simulink model "g4_regulated_converter"  (R2017a)
settings: Solver=ode23tb  StartTime=0  StopTime=1  RelTol=1e-3  EnableMultiTasking=on
undefined symbols (not defined in the file or in its folder): sigbuilder_block
libraries: powerlib x12, powerlib_meascontrol x1
settings Model: Creator=SHAKIL  LastModifiedBy=user
settings OptimizationCC: LifeSpan=inf
settings DebuggingCC: SFUnexpectedBacktrackingDiag=warning  SFNoUnconditionalDefaultTransitionDiag=warning  SFExecutionAtInitializationDiag=none
settings HardwareCC: ProdBitPerSizeT=32  ProdBitPerPtrDiffT=32  ProdWordSize=32  ProdHWDeviceType=Specified
settings GRTTargetCC: TargetLangStandard=C89/C90 (ANSI)  GeneratePreprocessorConditionals=Disable all
settings ConfigComp: CovMetricSettings=dw  CovHtmlReporting=on  CovSaveCumulativeToWorkspaceVar=on  CovSaveSingleToWorkspaceVar=on  CovExternalEMLEnable=off

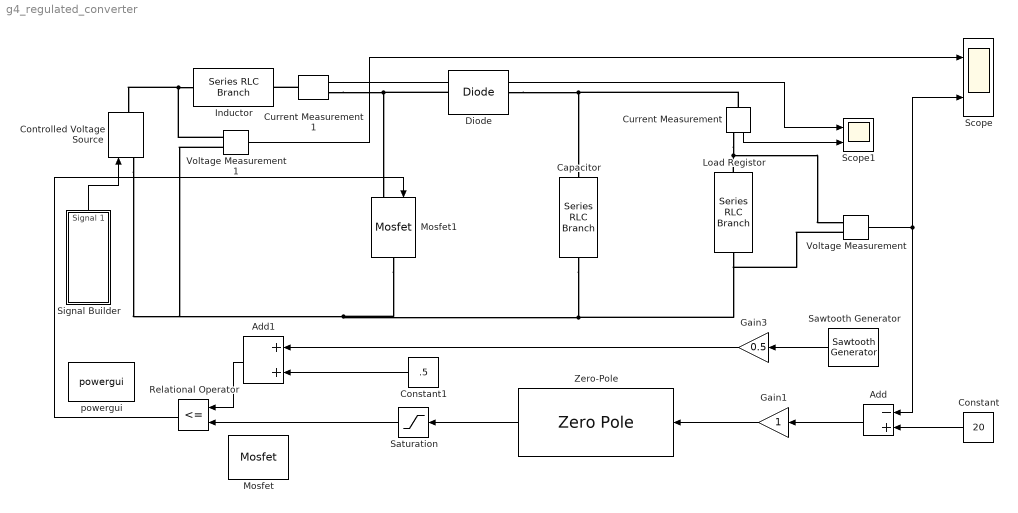
== system g4_regulated_converter ==
  Add : Sum  Inputs=-+
  Add1 : Sum
  Capacitor : powerlib/Elements/Series RLC Branch  LConnTagsString=__new0  RConnTagsString=__new0  BranchType=C  Resistance=1  Inductance=1e-3  SetiL0=off  InitialCurrent=0  Capacitance=78e-6  Setx0=off  InitialVoltage=0  Measurements=None
  Constant : Constant  Value=20
  Constant1 : Constant  Value=.5
  Controlled Voltage Source : powerlib/Electrical Sources/Controlled Voltage Source  Initialize=on  Source_Type=DC  Amplitude=0  Phase=0  Frequency=0  Measurements=None
  Current Measurement : powerlib/Measurements/Current Measurement  PhasorSimulation=off  OutputType=Complex  PSBequivalent=0
  Current Measurement1 : powerlib/Measurements/Current Measurement  PhasorSimulation=off  OutputType=Complex  PSBequivalent=0
  Diode : powerlib/Power Electronics/Diode  Ron=1e-9  Lon=0  Vf=0.1  IC=0  UseSnubber=off  Rs=0  Cs=0  Measurements=off
  Gain1 : Gain
  Gain3 : Gain  Gain=0.5
  Inductor : powerlib/Elements/Series RLC Branch  LConnTagsString=__new0  RConnTagsString=__new0  BranchType=L  Resistance=1  Inductance=35e-6  SetiL0=on  InitialCurrent=0  Capacitance=1e-6  Setx0=off  InitialVoltage=0  Measurements=None
  Load Registor : powerlib/Elements/Series RLC Branch  LConnTagsString=__new0  RConnTagsString=__new0  BranchType=R  Resistance=4  Inductance=1e-3  SetiL0=off  InitialCurrent=0  Capacitance=1e-6  Setx0=off  InitialVoltage=0  Measurements=None
  Mosfet : powerlib/Power Electronics/Mosfet  Ron=0.1  Lon=0  Rd=0.01  Vfd=0  IC=0  Rs=1e5  Cs=inf  Measurements=on
  Mosfet1 : powerlib/Power Electronics/Mosfet  Ron=0.1  Lon=0  Rd=0.01  Vfd=0  IC=0  Rs=1e5  Cs=inf  Measurements=off
  Relational Operator : RelationalOperator  Operator=<=  OutDataTypeStr=boolean  RndMeth=Nearest
  Saturation : Saturate  UpperLimit=0.6  LowerLimit=0.1
  Sawtooth Generator : powerlib_meascontrol/Pulse & Signal Generators/Sawtooth Generator  Freq=80e3  Phase=180  Ts=0
      settings: SourceProductName=Simscape Power Systems
  Scope : Scope  NumInputPorts=2
  Scope1 : Scope  NumInputPorts=2
  Signal Builder : Subsystem  Tag=STV Subsys  LoadFcn=sigbuilder_block('load');  StartFcn=sigbuilder_block('start');  StopFcn=sigbuilder_block('stop');  ClipboardFcn=sigbuilder_block('clipboard');  mask(Sigbuilder block){tuvar=[0:10]}
      mask help: Simulink:masks:SigbuilderBlock_MD
      mask init:
      | if ~strcmp(get_param(bdroot(gcbh),'SimulationStatus'),'stopped') tuvar = sigbuilder_block('maskInit'); end
      settings: CopyFcn=sigbuilder_block('copy');  DeleteFcn=sigbuilder_block('delete');  ModelCloseFcn=sigbuilder_block('modelClose');  PreSaveFcn=sigbuilder_block('preSave');  PauseFcn=sigbuilder_block('pause');  ContinueFcn=sigbuilder_block('continue');  NameChangeFcn=sigbuilder_block('namechange');  OpenFcn=sigbuilder_block('open',[6 6 1008 506.25 ]);  CloseFcn=sigbuilder_block('close');
      mask Display: plot(0, 0, 100, 100,[2, 2, 32, 32, 2], [68, 8, 8, 68, 68],[32, 2], [38, 38], [32, 19, 2],[53, 60, 44], [32, 17, 17, 2],[16, 16, 31, 31]);txt = getActiveGroup(gcbh);text(2, 100, txt,'verticalAlignment', 'top');
  Voltage Measurement : powerlib/Measurements/Voltage Measurement  PhasorSimulation=off  OutputType=Complex  PSBequivalent=0
  Voltage Measurement1 : powerlib/Measurements/Voltage Measurement  PhasorSimulation=off  OutputType=Complex  PSBequivalent=0
  Zero-Pole : ZeroPole  Zeros=[-2000 -2000]  Poles=[0 -10000]  Gain=[0.04]
  powergui : powerlib/powergui  Priority=1  SimulationMode=Continuous  SampleTime=50e-6  frequency=60  Iterations=50  frequencyindice=0  Pbase=100e6  ErrMax=1e-4  UnitsV=kV  UnitsW=MW  buscounter=0  FunctionMessages=off  echomessages=off  EnableUseOfTLC=off  CurrentSourceSwitches=off  DisableSnubberDevices=off  DisableRonSwitches=off  DisableVfSwitches=off  DisplayEquations=off  SolverType=Tustin/Backward Euler (TBE)  Interpol=off  ExternalGateDelay=off  methode=off  Ts=10  x0status=blocks  SPID=off  SwTol=0  HookPort=off  RestoreLinks=warning  ResistiveCurrentMeasurement=off  Frange=[0:2:500]  Ylog=off  Xlog=on  ShowGrid=off  save=off  variable=ZData  structure=0  ZoomFFT=off  StartTime=0.0  cycles=1  DisplayStyle=1  fundamental=60  FreqAxis=off  MaxFrequency=1000  frequencyindicesteady=1  RmsSteady=1  display=off
  wires:
  Voltage Measurement/1 -> Scope/2, Add/1
  Constant/1 -> Add/2
  Add/1 -> Gain1/1
  Signal Builder/1(Signal 1) -> Controlled Voltage Source/1
  Gain1/1 -> Zero-Pole/1
  Gain3/1 -> Add1/1
  Sawtooth Generator/1 -> Gain3/1
  Constant1/1 -> Add1/2
  Add1/1 -> Relational Operator/1
  Zero-Pole/1 -> Saturation/1
  Saturation/1 -> Relational Operator/2
  Voltage Measurement1/1 -> Scope/1
  Relational Operator/1 -> Mosfet1/1
  Current Measurement/1 -> Scope1/2
  Current Measurement1/1 -> Scope1/1
  connections:
  Voltage Measurement/LConn2 -- Load Registor/RConn1 -- Voltage Measurement1/LConn2 -- Controlled Voltage Source/LConn1 -- Mosfet1/RConn1 -- Capacitor/RConn1
  Load Registor/LConn1 -- Current Measurement/RConn1 -- Voltage Measurement/LConn1
  Diode/RConn1 -- Current Measurement/LConn1 -- Capacitor/LConn1
  Voltage Measurement1/LConn1 -- Controlled Voltage Source/RConn1 -- Inductor/LConn1
  Current Measurement1/LConn1 -- Inductor/RConn1
  Current Measurement1/RConn1 -- Mosfet1/LConn1 -- Diode/LConn1

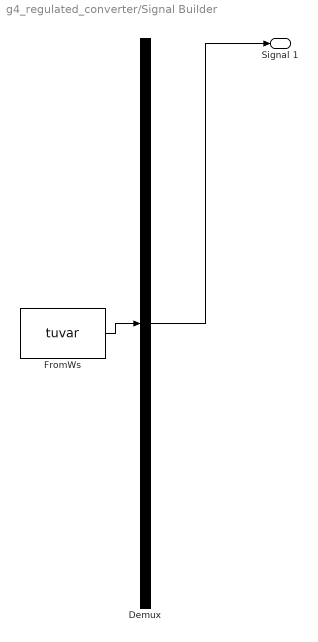
== system g4_regulated_converter/Signal Builder ==
  Demux : Demux  Tag=STV Demux  Outputs=1
  FromWs : FromWorkspace  Tag=STV FromWs  VariableName=tuvar  SampleTime=0
      SigBuilderData=|
      | common.afterFinalStr = 'Extrapolate'
      | common.sampleTime = 0
      | dataSet.timeRange = [0 10]
      | dataSet.name = 'Group 1'
      | sbobj.Groups.Name = 'Group 1'
      | sbobj.Groups.Signals.Name = 'Signal 1'
      | sbobj.Groups.Signals.XData = [0 0.1 0.1 0.33 0.33 0.557 0.557 0.728 0.728 2.02 2.02 10]
      | sbobj.Groups.Signals.YData = [15 15 13.9 13.9 12.74 12.74 11.88 11.88 14.7 14.7 15 15]
  Signal 1 : Outport  Tag=STV Outport
  wires:
  Demux/1 -> Signal 1/1
  FromWs/1 -> Demux/1
